simulink model "VELOCIDAD"  (R2015a)
settings: Solver=ode3  SolverMode=SingleTasking  StartTime=0.0  StopTime=inf  RelTol=1e-3
InitFcn:
  | % Periodo de muestreo control
  | %ts=5e-3;
  | % Periodo de muestreo control logico
  | tc=ts;
  | % Periodo de muestreo registro
  | tr=5e-3;
  | % Radio de la rueda (m)
  | R=86.1e-3/2;
  | % Distancia entre ruedas (m)
  | W=0.160;
  | % Constante de tiempo de filtrado
  | Tf_vel=200e-3; % Velocidad
values from neighbouring files (symbols this model uses):
  Cd = K*(1+1/(Ti*sd)+(Td*sd)/(1+Td*sd/N))    [ControlP.m]    (also in dead_2015.m = minreal(Fd/Pd/(1-Fd)); p4_3_diseño_directo.m = minreal(F/(Pd-F*Pd)))
  Crd = Cd    [ControlP.m]    (also in dead_2015.m; p4_3_diseño_directo.m)
  ts = 0.5    [ControlP.m]    (also in ControlPID_RF.m = 0.005; dead_2015.m = 0.055)
libraries: legonxtlib x6, simulink x3
settings Model: SimulationMode=external  CovSFcnEnable=off  ExtModeTrigDuration=2  Creator=mogimenez  LastModifiedBy=stic
settings DataIOCC: SignalLoggingSaveFormat=ModelDataLogs
settings OptimizationCC: ExpressionDepthLimit=2147483647  OptimizeModelRefInitCode=on  LifeSpan=1
settings DebuggingCC: UnderspecifiedInitializationDetection=Classic  MergeDetectMultiDrivingBlocksExec=none  ParameterPrecisionLossMsg=none  FcnCallInpInsideContextMsg=EnableAllAsWarning  StateNameClashWarn=warning
settings HardwareCC: ProdLargestAtomicInteger=Long  ProdLargestAtomicFloat=Float  ProdEndianess=LittleEndian  ProdHWDeviceType=ARM Compatible->ARM 7
settings RTWCC: SystemTargetFile=realtime.tlc  GenerateMakefile=off  TemplateMakefile=realtime.tmf  Description=Real-Time Toolbox  RTWVerbose=off
settings CodeAppCC: CustomSymbolStrType=$N$R$M  InternalIdentifier=Classic
settings ERTTargetCC: CombineOutputUpdateFcns=off  ExtMode=on  ExtModeTransport=1  ExtModeMexArgs=0 4 9600  InlinedParameterPlacement=Hierarchical  ERTSrcFileBannerTemplate=realtime_code_template.cgt  ERTHdrFileBannerTemplate=realtime_code_template.cgt  ERTDataSrcFileTemplate=realtime_code_template.cgt  ERTDataHdrFileTemplate=realtime_code_template.cgt  ERTCustomFileTemplate=realtime_file_process.tlc

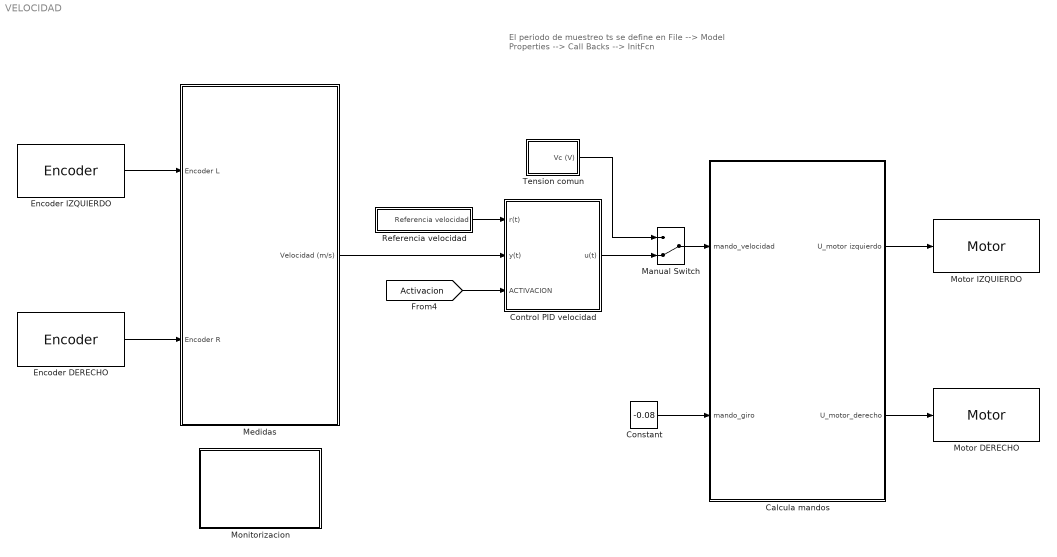
== system VELOCIDAD ==
  note: El periodo de muestreo ts se define en
      | File --> Model Properties --> Call Backs --> InitFcn
  Calcula mandos : Subsystem
  Constant : Constant  Value=-0.08  SampleTime=ts
  Control PID velocidad : Subsystem
  Encoder DERECHO : legonxtlib/Encoder  portNumber=C  opMode=No reset  sampleTime=tr  blockPlatform=LegoMindstormsNXT
  Encoder IZQUIERDO : legonxtlib/Encoder  portNumber=B  opMode=No reset  sampleTime=tr  blockPlatform=LegoMindstormsNXT
  Manual Switch : ManualSwitch  CurrentSetting=0
  Medidas : Subsystem
  Monitorizacion : Subsystem
  Motor DERECHO : legonxtlib/Motor  sportNumber=C  sstopAction=Brake  blockPlatform=LegoMindstormsNXT
  Motor IZQUIERDO : legonxtlib/Motor  sportNumber=B  sstopAction=Brake  blockPlatform=LegoMindstormsNXT
  Referencia velocidad : Subsystem  mask{Vmax=0.15, Vmin=0.1, T=2}
      mask prompts: Vmax "Valor maximo"; Vmin "Valor minimo"; T "Periodo (s)"
  Tension comun : Subsystem
  wires:
  Encoder DERECHO/1 -> Medidas/2(Encoder R)
  [Activacion] -> Control PID velocidad/3(ACTIVACION)
  Constant/1 -> Calcula mandos/2(mando_giro)
  Calcula mandos/1(U_motor izquierdo) -> Motor IZQUIERDO/1
  Calcula mandos/2(U_motor_derecho) -> Motor DERECHO/1
  Referencia velocidad/1(Referencia velocidad) -> Control PID velocidad/1(r(t))
  Medidas/1(Velocidad (m/s)) -> Control PID velocidad/2(y(t))
  Encoder IZQUIERDO/1 -> Medidas/1(Encoder L)
  Tension comun/1(Vc (V)) -> Manual Switch/1
  Manual Switch/1 -> Calcula mandos/1(mando_velocidad)
  Control PID velocidad/1(u(t)) -> Manual Switch/2

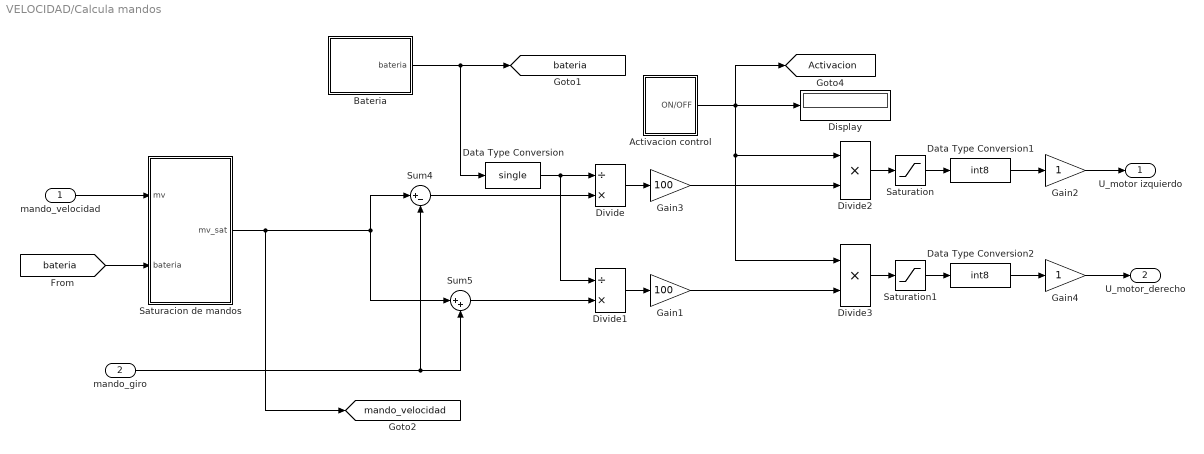
== system VELOCIDAD/Calcula mandos ==
  mando_velocidad : Inport
  mando_giro : Inport  Port=2
  Activacion control : Subsystem
  Bateria : Subsystem
  Data Type Conversion : DataTypeConversion  OutDataTypeStr=single  SampleTime=ts
  Data Type Conversion1 : DataTypeConversion  OutDataTypeStr=int8
  Data Type Conversion2 : DataTypeConversion  OutDataTypeStr=int8
  Display : Display
  Divide : Product  Inputs=/*
  Divide1 : Product  Inputs=/*
  Divide2 : Product  SampleTime=ts
  Divide3 : Product  SampleTime=ts
  Gain1 : Gain  Gain=100
  Gain2 : Gain
  Gain3 : Gain  Gain=100
  Gain4 : Gain
  Saturacion de mandos : Subsystem
  Saturation : Saturate  UpperLimit=100  LowerLimit=-100
  Saturation1 : Saturate  UpperLimit=100  LowerLimit=-100
  Sum4 : Sum  Inputs=|+-
  Sum5 : Sum  Inputs=|++
  U_motor izquierdo : Outport
  U_motor_derecho : Outport  Port=2
  tag scope: Activacion=global, bateria=global, mando_velocidad=global
  wires:
  Divide/1 -> Gain3/1
  Sum4/1 -> Divide/2
  Divide1/1 -> Gain1/1
  Sum5/1 -> Divide1/2
  mando_giro/1 -> Sum4/2, Sum5/2
  Bateria/1(bateria) -> Data Type Conversion/1, [bateria]
  Divide2/1 -> Saturation/1
  Divide3/1 -> Saturation1/1
  Activacion control/1(ON/OFF) -> Display/1, Divide2/1, Divide3/1, [Activacion]
  Data Type Conversion1/1 -> Gain2/1
  Data Type Conversion2/1 -> Gain4/1
  Data Type Conversion/1 -> Divide/1, Divide1/1
  Saturation/1 -> Data Type Conversion1/1
  Saturation1/1 -> Data Type Conversion2/1
  [bateria] -> Saturacion de mandos/2(bateria)
  Gain3/1 -> Divide2/2
  Gain1/1 -> Divide3/2
  mando_velocidad/1 -> Saturacion de mandos/1(mv)
  Gain2/1 -> U_motor izquierdo/1
  Gain4/1 -> U_motor_derecho/1
  Saturacion de mandos/1(mv_sat) -> [mando_velocidad], Sum4/1, Sum5/1

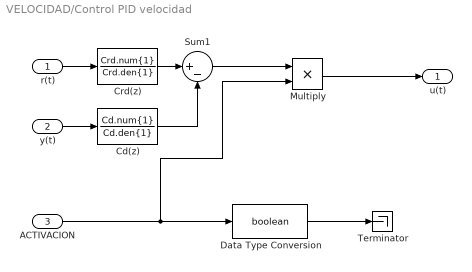
== system VELOCIDAD/Control PID velocidad ==
  r(t) : Inport  SampleTime=ts
  y(t) : Inport  Port=2  SampleTime=ts
  ACTIVACION : Inport  Port=3  SampleTime=ts
  Cd(z) : DiscreteTransferFcn  Numerator=Cd.num{1}  Denominator=Cd.den{1}  SampleTime=ts
  "Crd(z) " : DiscreteTransferFcn  Numerator=Crd.num{1}  Denominator=Crd.den{1}  SampleTime=ts
  Data Type Conversion : DataTypeConversion  OutDataTypeStr=boolean
  Multiply : Product  Inputs=**
  Sum1 : Sum  Inputs=|+-
  Terminator : Terminator
  u(t) : Outport
  wires:
  ACTIVACION/1 -> Multiply/2, Data Type Conversion/1
  Data Type Conversion/1 -> Terminator/1
  r(t)/1 -> "Crd(z) "/1
  "Crd(z) "/1 -> Sum1/1
  Cd(z)/1 -> Sum1/2
  y(t)/1 -> Cd(z)/1
  Sum1/1 -> Multiply/1
  Multiply/1 -> u(t)/1

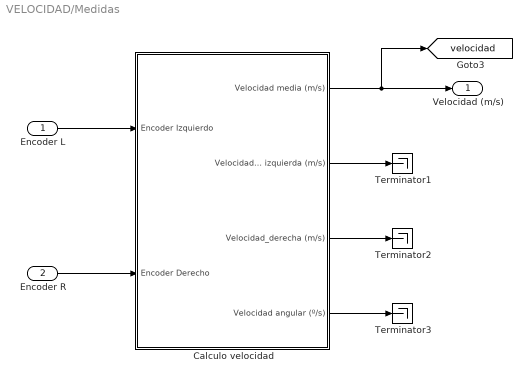
== system VELOCIDAD/Medidas ==
  Encoder L : Inport
  Encoder R : Inport  Port=2
  Calculo velocidad : Subsystem
  Terminator1 : Terminator
  Terminator2 : Terminator
  Terminator3 : Terminator
  Velocidad (m/s) : Outport
  tag scope: velocidad=global
  wires:
  Encoder R/1 -> Calculo velocidad/2(Encoder Derecho)
  Encoder L/1 -> Calculo velocidad/1(Encoder Izquierdo)
  Calculo velocidad/1(Velocidad media (m/s)) -> Velocidad (m/s)/1, [velocidad]
  Calculo velocidad/4(Velocidad angular (º/s)) -> Terminator3/1
  Calculo velocidad/2(Velocidad izquierda (m/s)) -> Terminator1/1
  Calculo velocidad/3(Velocidad_derecha (m/s)) -> Terminator2/1

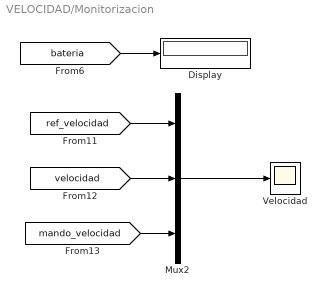
== system VELOCIDAD/Monitorizacion ==
  Display : Display
  Mux2 : Mux  Inputs=3
  Velocidad : Scope
      settings: TimeRange=10  YMin=-4.5  YMax=6  SaveName=Velocidad  SampleInput=on  SampleTime=tr
  wires:
  [bateria] -> Display/1
  [ref_velocidad] -> Mux2/1
  [mando_velocidad] -> Mux2/3
  [velocidad] -> Mux2/2
  Mux2/1 -> Velocidad/1

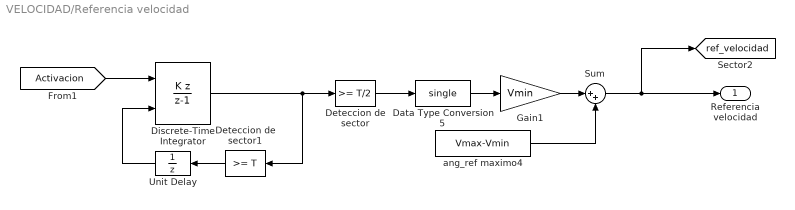
== system VELOCIDAD/Referencia velocidad ==
  Data Type Conversion5 : DataTypeConversion  OutDataTypeStr=single
  Deteccion de sector : simulink/Logic and Bit Operations/Compare To Constant  relop=>=  const=T/2  OutDataTypeStr=uint8
  Deteccion de sector1 : simulink/Logic and Bit Operations/Compare To Constant  relop=>=  const=T  OutDataTypeStr=uint8
  Discrete-Time Integrator : DiscreteIntegrator  IntegratorMethod=Accumulation: Backward Euler  gainval=tc  ExternalReset=rising  SampleTime=tc  OutDataTypeStr=single  UpperSaturationLimit=10  LowerSaturationLimit=0
  Gain1 : Gain  Gain=Vmin  ParamDataTypeStr=double  OutDataTypeStr=single
  Sum : Sum  Inputs=|++  SampleTime=ts
  Unit Delay : UnitDelay  SampleTime=tc
  ang_ref maximo4 : Constant  Value=Vmax-Vmin  OutDataTypeStr=single  SampleTime=tc
  Referencia velocidad : Outport  SampleTime=ts
  tag scope: ref_velocidad=global
  wires:
  ang_ref maximo4/1 -> Sum/2
  [Activacion] -> Discrete-Time Integrator/1
  Discrete-Time Integrator/1 -> Deteccion de sector1/1, Deteccion de sector/1
  Deteccion de sector/1 -> Data Type Conversion5/1
  Unit Delay/1 -> Discrete-Time Integrator/2
  Data Type Conversion5/1 -> Gain1/1
  Gain1/1 -> Sum/1
  Deteccion de sector1/1 -> Unit Delay/1
  Sum/1 -> [ref_velocidad], Referencia velocidad/1

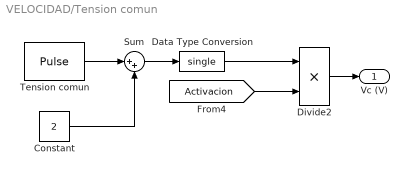
== system VELOCIDAD/Tension comun ==
  Constant : Constant  Value=2
  Data Type Conversion : DataTypeConversion  OutDataTypeStr=single
  Divide2 : Product  SampleTime=ts
  Sum : Sum  Inputs=|++
  Tension comun : DiscretePulseGenerator  Amplitude=2  Period=floor(1/ts)  PulseWidth=floor(0.5/ts)  SampleTime=ts
  Vc (V) : Outport
  wires:
  Tension comun/1 -> Sum/1
  Sum/1 -> Data Type Conversion/1
  Constant/1 -> Sum/2
  Divide2/1 -> Vc (V)/1
  Data Type Conversion/1 -> Divide2/1
  [Activacion] -> Divide2/2

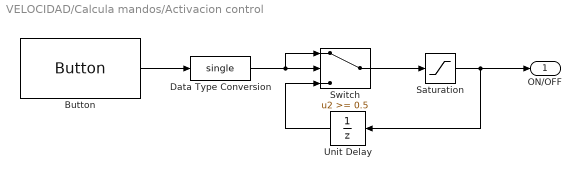
== system VELOCIDAD/Calcula mandos/Activacion control ==
  Button : legonxtlib/Button  buttonType=Middle orange  sampleTime=tc  blockPlatform=LegoMindstormsNXT
  Data Type Conversion : DataTypeConversion  OutDataTypeStr=single
  Saturation : Saturate  UpperLimit=1  LowerLimit=0
  Switch : Switch  Threshold=0.5
  Unit Delay : UnitDelay  SampleTime=tc
  ON/OFF : Outport
  wires:
  Button/1 -> Data Type Conversion/1
  Switch/1 -> Saturation/1
  Unit Delay/1 -> Switch/3
  Data Type Conversion/1 -> Switch/2, Switch/1
  Saturation/1 -> Unit Delay/1, ON/OFF/1

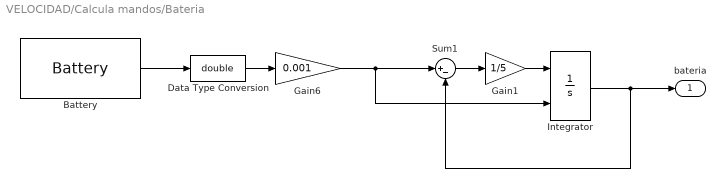
== system VELOCIDAD/Calcula mandos/Bateria ==
  Battery : legonxtlib/Battery  sampleTime=0.1  blockPlatform=LegoMindstormsNXT
  Data Type Conversion : DataTypeConversion  OutDataTypeStr=double
  Gain1 : Gain  Gain=1/5
  Gain6 : Gain  Gain=0.001
  Integrator : Integrator  InitialConditionSource=external
  Sum1 : Sum  Inputs=|+-
  bateria : Outport
  wires:
  Battery/1 -> Data Type Conversion/1
  Data Type Conversion/1 -> Gain6/1
  Sum1/1 -> Gain1/1
  Integrator/1 -> bateria/1, Sum1/2
  Gain6/1 -> Sum1/1, Integrator/2
  Gain1/1 -> Integrator/1

== system VELOCIDAD/Calcula mandos/Saturacion de mandos ==
  mv : Inport
  bateria : Inport  Port=2  SampleTime=ts
  Gain8 : Gain  Gain=-1
  Saturation Dynamic : simulink/Discontinuities/Saturation Dynamic  OutMin=[]  OutMax=[]  OutDataTypeStr=Inherit: Same as second input  OutDataType=fixdt(1, 16)  OutScaling=2^-10  DoSatur=off
  mv_sat : Outport
  wires:
  Gain8/1 -> Saturation Dynamic/3
  bateria/1 -> Gain8/1, Saturation Dynamic/1
  mv/1 -> Saturation Dynamic/2
  Saturation Dynamic/1 -> mv_sat/1

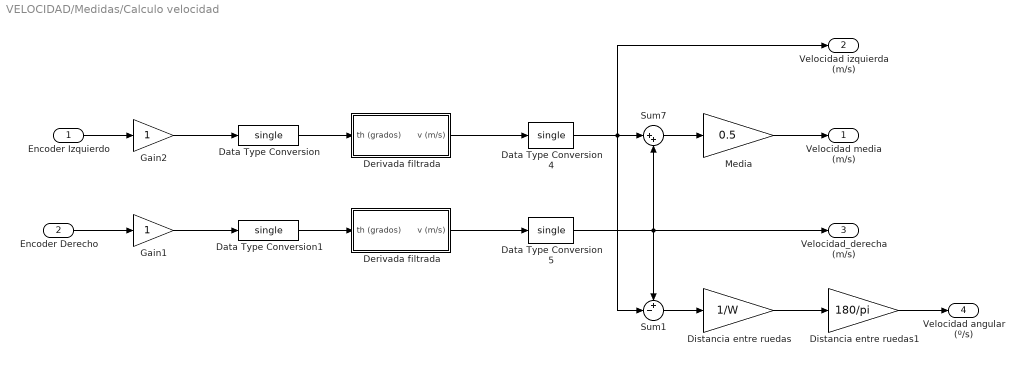
== system VELOCIDAD/Medidas/Calculo velocidad ==
  Encoder Izquierdo : Inport
  Encoder Derecho : Inport  Port=2
  Data Type Conversion{,1,4..5} (4 alike) : DataTypeConversion  OutDataTypeStr=single
  Derivada filtrada : Subsystem  mask{R=R, T=Tf_vel, ts=tr}
      mask prompts: R "Radio rueda (m)"; T "Constante de tiempo filtrado (s)"; ts "Periodo de muestreo"
      mask init:
      | alfa=exp(-ts/T);
  "Derivada filtrada " : Subsystem  mask{R=R, T=Tf_vel, ts=tr}
      mask prompts: R "Radio rueda (m)"; T "Constante de tiempo filtrado (s)"; ts "Periodo de muestreo"
      mask init:
      | alfa=exp(-ts/T);
  Distancia entre ruedas : Gain  Gain=1/W
  Distancia entre ruedas1 : Gain  Gain=180/pi
  Gain1 : Gain
  Gain2 : Gain
  Media : Gain  Gain=0.5
  Sum1 : Sum  Inputs=+-|
  Sum7 : Sum  Inputs=|++
  Velocidad media (m/s) : Outport
  Velocidad izquierda (m/s) : Outport  Port=2
  Velocidad_derecha (m/s) : Outport  Port=3
  Velocidad angular (º/s) : Outport  Port=4
  wires:
  Data Type Conversion1/1 -> Derivada filtrada/1(th (grados))
  Derivada filtrada/1(v (m/s)) -> Data Type Conversion5/1
  "Derivada filtrada "/1(v (m/s)) -> Data Type Conversion4/1
  Encoder Izquierdo/1 -> Gain2/1
  Data Type Conversion4/1 -> Sum1/2, Velocidad izquierda (m/s)/1, Sum7/1
  Encoder Derecho/1 -> Gain1/1
  Data Type Conversion5/1 -> Sum1/1, Velocidad_derecha (m/s)/1, Sum7/2
  Sum7/1 -> Media/1
  Media/1 -> Velocidad media (m/s)/1
  Data Type Conversion/1 -> "Derivada filtrada "/1(th (grados))
  Sum1/1 -> Distancia entre ruedas/1
  Distancia entre ruedas/1 -> Distancia entre ruedas1/1
  Distancia entre ruedas1/1 -> Velocidad angular (º/s)/1
  Gain2/1 -> Data Type Conversion/1
  Gain1/1 -> Data Type Conversion1/1

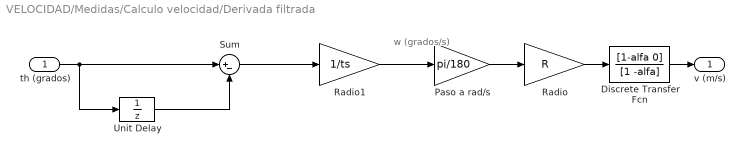
== system VELOCIDAD/Medidas/Calculo velocidad/Derivada filtrada ==
  note: w (grados/s)
  th (grados) : Inport  SampleTime=ts
  Discrete Transfer Fcn : DiscreteTransferFcn  Numerator=[1-alfa 0]  Denominator=[1 -alfa]
  Paso a rad/s : Gain  Gain=pi/180
  Radio : Gain  Gain=R
  Radio1 : Gain  Gain=1/ts
  Sum : Sum  Inputs=|+-
  Unit Delay : UnitDelay  SampleTime=-1
  v (m/s) : Outport
  wires:
  th (grados)/1 -> Unit Delay/1, Sum/1
  Unit Delay/1 -> Sum/2
  Sum/1 -> Radio1/1
  Radio1/1 -> Paso a rad/s/1
  Paso a rad/s/1 -> Radio/1
  Radio/1 -> Discrete Transfer Fcn/1
  Discrete Transfer Fcn/1 -> v (m/s)/1

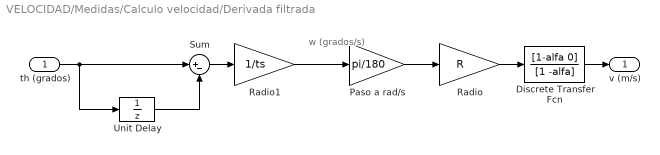
== system VELOCIDAD/Medidas/Calculo velocidad/Derivada filtrada  ==
  note: w (grados/s)
  th (grados) : Inport  SampleTime=ts
  Discrete Transfer Fcn : DiscreteTransferFcn  Numerator=[1-alfa 0]  Denominator=[1 -alfa]
  Paso a rad/s : Gain  Gain=pi/180
  Radio : Gain  Gain=R
  Radio1 : Gain  Gain=1/ts
  Sum : Sum  Inputs=|+-
  Unit Delay : UnitDelay  SampleTime=-1
  v (m/s) : Outport
  wires:
  Discrete Transfer Fcn/1 -> v (m/s)/1
  Radio/1 -> Discrete Transfer Fcn/1
  Paso a rad/s/1 -> Radio/1
  Radio1/1 -> Paso a rad/s/1
  Sum/1 -> Radio1/1
  Unit Delay/1 -> Sum/2
  th (grados)/1 -> Sum/1, Unit Delay/1
